simulink model "p4"  (R2021b)
settings: Solver=VariableStepAuto  StartTime=0.0  StopTime=30.0  RelTol=1e-3
settings Model: Creator=mahya  LastModifiedBy=mahya

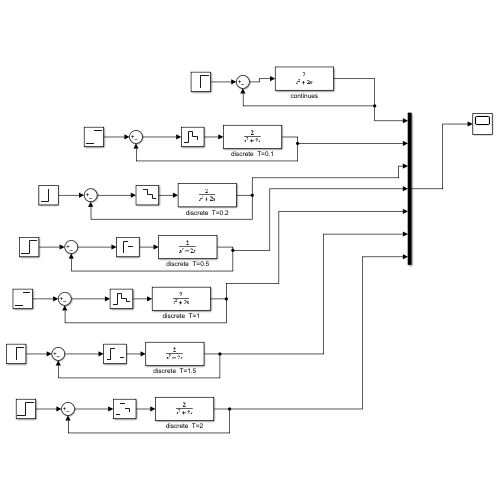
[thumbnail: Simulink's stored preview of the top-level diagram]
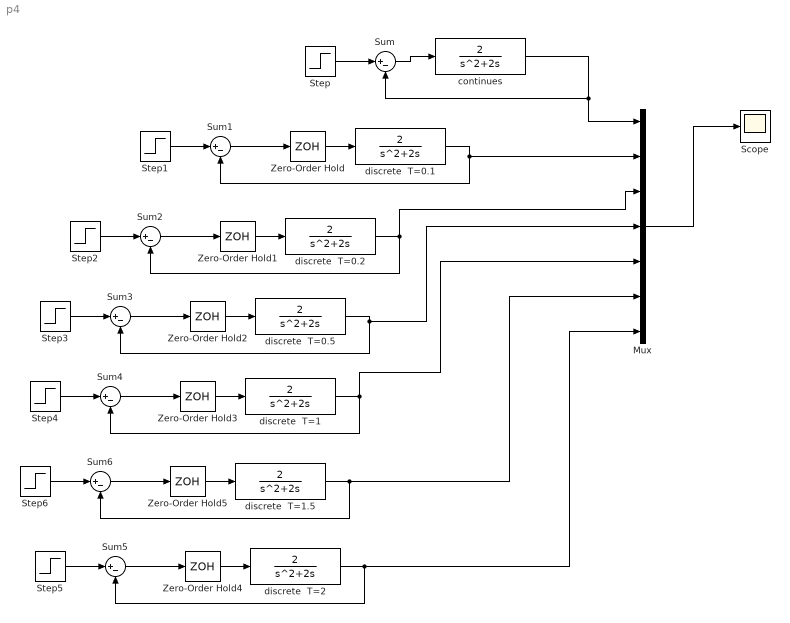
== system p4 ==
  Mux : Mux  Inputs=7
  Scope : Scope
  Step{,1..6} (7 alike) : Step  Time=0  SampleTime=0
  Sum{,1..6} (7 alike) : Sum  Inputs=|+-
  Zero-Order Hold : ZeroOrderHold  SampleTime=0.1
  Zero-Order Hold1 : ZeroOrderHold  SampleTime=0.2
  Zero-Order Hold2 : ZeroOrderHold  SampleTime=0.5
  Zero-Order Hold3 : ZeroOrderHold
  Zero-Order Hold4 : ZeroOrderHold  SampleTime=2
  Zero-Order Hold5 : ZeroOrderHold  SampleTime=1.5
  continues : TransferFcn  Numerator=[2]  Denominator=[ 1 2 0]
  discrete  T=0.1 : TransferFcn  Numerator=[2]  Denominator=[ 1 2 0]
  discrete  T=0.2 : TransferFcn  Numerator=[2]  Denominator=[ 1 2 0]
  discrete  T=0.5 : TransferFcn  Numerator=[2]  Denominator=[ 1 2 0]
  discrete  T=1 : TransferFcn  Numerator=[2]  Denominator=[ 1 2 0]
  discrete  T=1.5 : TransferFcn  Numerator=[2]  Denominator=[ 1 2 0]
  discrete  T=2 : TransferFcn  Numerator=[2]  Denominator=[ 1 2 0]
  wires:
  continues/1 -> Mux/1, Sum/2
  Step/1 -> Sum/1
  Sum/1 -> continues/1
  Step1/1 -> Sum1/1
  discrete  T=0.1/1 -> Mux/2, Sum1/2
  Sum1/1 -> Zero-Order Hold/1
  Zero-Order Hold/1 -> discrete  T=0.1/1
  Mux/1 -> Scope/1
  Step2/1 -> Sum2/1
  discrete  T=0.2/1 -> Sum2/2, Mux/3
  Sum2/1 -> Zero-Order Hold1/1
  Zero-Order Hold1/1 -> discrete  T=0.2/1
  Sum3/1 -> Zero-Order Hold2/1
  Step3/1 -> Sum3/1
  discrete  T=0.5/1 -> Mux/4, Sum3/2
  Zero-Order Hold2/1 -> discrete  T=0.5/1
  Sum4/1 -> Zero-Order Hold3/1
  Step4/1 -> Sum4/1
  Zero-Order Hold3/1 -> discrete  T=1/1
  discrete  T=1/1 -> Mux/5, Sum4/2
  Zero-Order Hold4/1 -> discrete  T=2/1
  Step5/1 -> Sum5/1
  Sum5/1 -> Zero-Order Hold4/1
  discrete  T=2/1 -> Mux/7, Sum5/2
  Zero-Order Hold5/1 -> discrete  T=1.5/1
  Step6/1 -> Sum6/1
  Sum6/1 -> Zero-Order Hold5/1
  discrete  T=1.5/1 -> Mux/6, Sum6/2
